simulink model "Retro_de_estados_simulink"  (R2020a)
settings: Solver=VariableStepAuto  StartTime=0.0  StopTime=10.0  RelTol=1e-3
undefined symbols (not defined in the file): bm, g, K, K_motor, Ki, kr, L, m_total, R
settings Model: Creator=Noxi-PC  LastModifiedBy=Noxi-PC

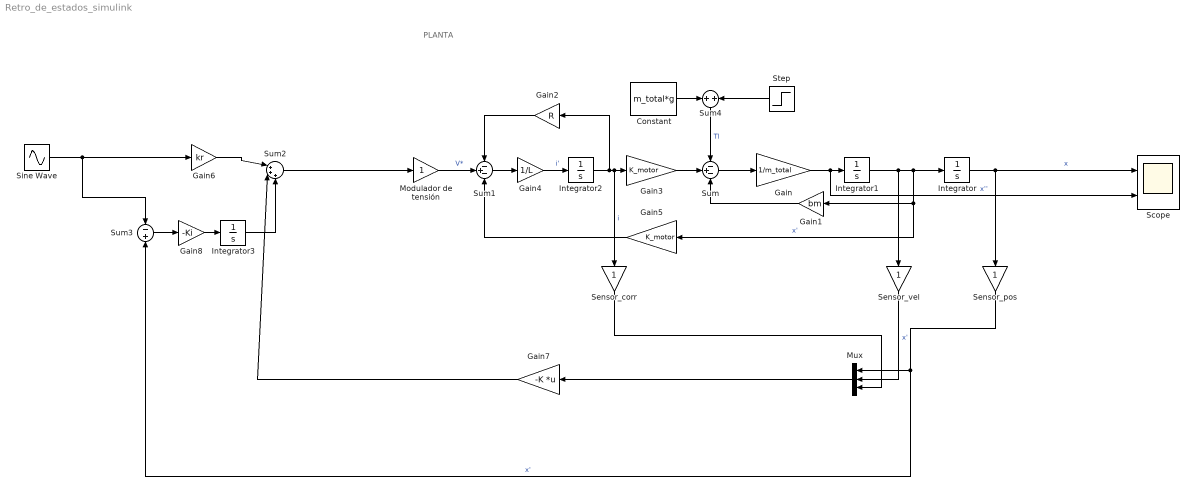
== system Retro_de_estados_simulink ==
  note: PLANTA
  " Sensor_pos" : Gain
  " Sensor_vel" : Gain
  Constant : Constant  Value=m_total*g
  Gain : Gain  Gain=1/m_total
  Gain1 : Gain  Gain=bm
  Gain2 : Gain  Gain=R
  Gain3 : Gain  Gain=K_motor
  Gain4 : Gain  Gain=1/L
  Gain5 : Gain  Gain=K_motor
  Gain6 : Gain  Gain=kr
  Gain7 : Gain  Gain=-K  Multiplication=Matrix(K*u)
  Gain8 : Gain  Gain=-Ki
  Integrator{,1..3} (4 alike) : Integrator
  Modulador de tensión : Gain
  Mux : Mux  Inputs=3
  Scope : Scope  NumInputPorts=2
  Sensor_corr : Gain
  Sine Wave : Sin  Frequency=10  SampleTime=0
  Step : Step  Time=3  After=0  SampleTime=0
  Sum : Sum  Inputs=-+-
  Sum1 : Sum  Inputs=-+-
  Sum2 : Sum  Inputs=|+++
  Sum3 : Sum  Inputs=-+
  Sum4 : Sum
  wires:
  Constant/1 -> Sum4/1
  Gain5/1 -> Sum1/3
  Gain1/1 -> Sum/3
  Integrator2/1 -> Gain2/1, Gain3/1, Sensor_corr/1  "i"
  Sum4/1 -> Sum/1  "Tl"
  Modulador de tensión/1 -> Sum1/2  "V*"
  Sum/1 -> Gain/1
  Step/1 -> Sum4/2
  Sum1/1 -> Gain4/1
  Gain4/1 -> Integrator2/1  "i'"
  Gain2/1 -> Sum1/1
  Gain3/1 -> Sum/2
  Gain/1 -> Scope/2, Integrator1/1  "x''"
  Integrator1/1 -> " Sensor_vel"/1, Gain5/1, Gain1/1, Integrator/1  "x'"
  Integrator/1 -> " Sensor_pos"/1, Scope/1  "x"
  Sum2/1 -> Modulador de tensión/1
  Sine Wave/1 -> Sum3/1, Gain6/1
  Gain6/1 -> Sum2/1
  " Sensor_pos"/1 -> Sum3/2, Mux/1  "x'"
  " Sensor_vel"/1 -> Mux/2  "x'"
  Sensor_corr/1 -> Mux/3
  Mux/1 -> Gain7/1
  Gain7/1 -> Sum2/2
  Sum3/1 -> Gain8/1
  Gain8/1 -> Integrator3/1
  Integrator3/1 -> Sum2/3
